simulink model "Model_XInput_wFeedback"  (R2023a)
settings: Solver=FixedStepAuto  StartTime=0.0  StopTime=100  FixedStep=0.01  RelTol=1e-3
settings Model: Creator=Mathias Voigt  LastModifiedBy=FIRSTMentor
settings SolverCC: AlgebraicLoopSolver=TrustRegion
settings DebuggingCC: UnconnectedInputMsg=warning  UnconnectedOutputMsg=warning  UnconnectedLineMsg=warning
settings ModelReferenceCC: EnableRefExpFcnMdlSchedulingChecks=on
settings SFSimCC: CustomCodeUndefinedFunction=UseInterfaceOnly

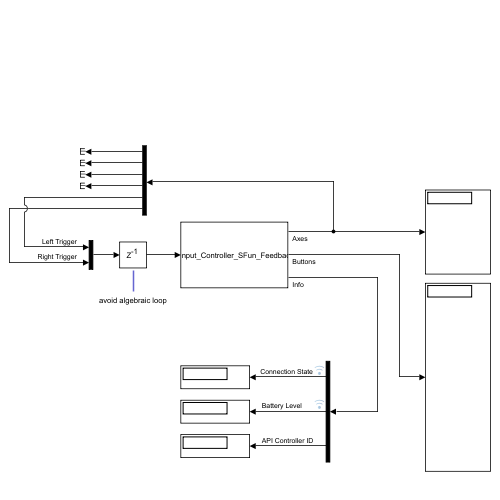
[thumbnail: Simulink's stored preview of the top-level diagram]
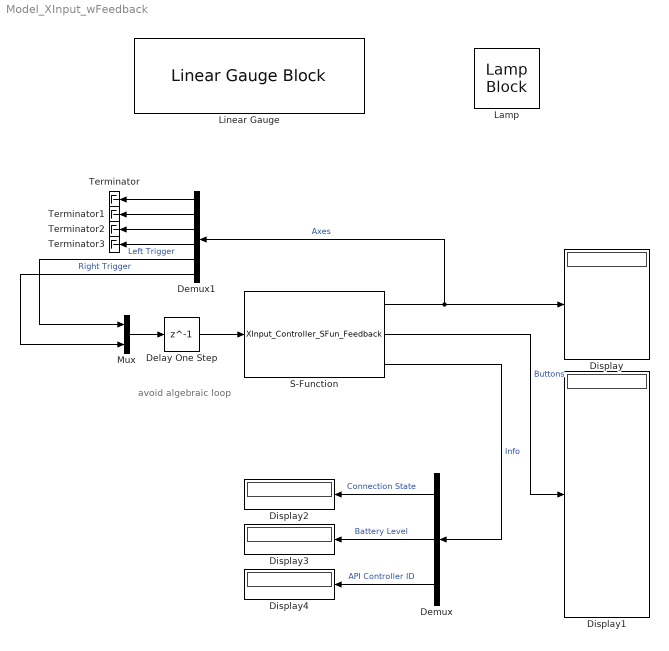
== system Model_XInput_wFeedback ==
  note: avoid algebraic loop
  Delay One Step : Delay  DelayLength=1
  Demux : Demux  Outputs=3
  Demux1 : Demux  Outputs=6
  Display{,1..4} (5 alike) : Display
  Lamp : LampBlock
  Linear Gauge : LinearGaugeBlock  TickInterval=25
  Mux : Mux  Inputs=2
  S-Function : S-Function  FunctionName=XInput_Controller_SFun_Feedback  Parameters=1  SFunctionDeploymentMode=off  EnableBusSupport=off
  Terminator{,1..3} (4 alike) : Terminator
  wires:
  S-Function/2 -> Display1/1  "Buttons"
  S-Function/1 -> Demux1/1, Display/1  "Axes"
  Demux/1 -> Display2/1  "Connection State"
  Demux/2 -> Display3/1  "Battery Level"
  Demux/3 -> Display4/1  "API Controller ID"
  S-Function/3 -> Demux/1  "Info"
  Delay One Step/1 -> S-Function/1
  Mux/1 -> Delay One Step/1
  Demux1/6 -> Mux/2  "Right Trigger"
  Demux1/5 -> Mux/1  "Left Trigger"
  Demux1/1 -> Terminator/1
  Demux1/2 -> Terminator1/1
  Demux1/3 -> Terminator2/1
  Demux1/4 -> Terminator3/1
